simulink model "controladorpruebaio2"  (R2025a)
settings: Solver=FixedStepAuto  StartTime=0.0  StopTime=inf  FixedStep=0.015  RelTol=1e-3  EnableMultiTasking=on
libraries: px4Peripheralslib x1, px4uORBlib x1
settings Model: PacingRate=0.790000  ExtModeTrigDuration=10  Creator=The MathWorks, Inc.  LastModifiedBy=aero
settings SolverCC: AlgebraicLoopSolver=TrustRegion  PositivePriorityOrder=on  AutoInsertRateTranBlk=on  MaxZcPerStep=1.0
settings OptimizationCC: EnhancedBackFolding=on  PassReuseOutputArgsAs=Individual arguments  MaxStackSize=64  OptimizeBlockOrder=speed  DifferentSizesBufferReuse=on  OptimizationCustomize=off  EfficientTunableParamExpr=on
settings DebuggingCC: ParameterPrecisionLossMsg=none  ParameterTunabilityLossMsg=error  UnconnectedInputMsg=warning  UnconnectedOutputMsg=warning  UnconnectedLineMsg=warning  SubsystemReferenceDiagnosticForUnitTest=warning  ArithmeticOperatorsInVariantConditions=warning
settings HardwareCC: ProdBitPerPointer=32.0  ProdBitPerSizeT=32.0  ProdBitPerPtrDiffT=32.0  ProdLargestAtomicInteger=Long  ProdLargestAtomicFloat=Double  ProdWordSize=32.0  ProdLongLongMode=on  ProdHWDeviceType=ARM Compatible->ARM Cortex
settings ModelReferenceCC: EnableRefExpFcnMdlSchedulingChecks=on
settings SFSimCC: MATLABDynamicMemAlloc=off  SimTargetLang=C++  SimDLTargetLibrary=mkl-dnn
settings RTWCC: SystemTargetFile=ert.tlc  HardwareBoard=PX4 Pixhawk 6c  TLCOptions="-aInlineSetEventsForThisBaseRateFcn=TLC_FALSE -aSuppressMultiTaskScheduler=TLC_FALSE  -aRateBasedStepFcn=0"  TemplateMakefile=ert_default_tmf  GenerateReport=on  Toolchain=GNU Tools for PX4 Autopilots  IncludeHyperlinkInReport=on  LaunchReport=on  TargetLang=C++  GenerateTraceInfo=on  GenerateTraceReport=on  GenerateTraceReportSl=on  GenerateTraceReportSf=on  GenerateTraceReportEml=on  GPUComputeCapability=3.5  DLArmComputeVersion=19.05  Description=Embedded Coder
settings CodeAppCC: ForceParamTrailComments=on  IgnoreCustomStorageClasses=off  OperatorAnnotations=on  SimulinkDataObjDesc=on  SFDataObjDesc=on  InsertBlockDesc=on
settings ERTTargetCC: ExtModeTransport=3.0  ExtModeStaticAllocSize=1024.0  InlinedParameterPlacement=Hierarchical

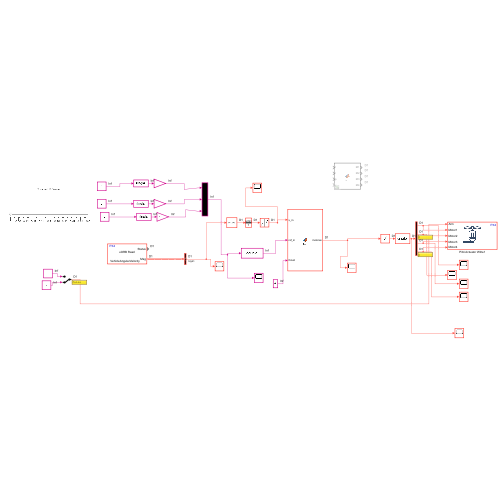
[thumbnail: Simulink's stored preview of the top-level diagram]
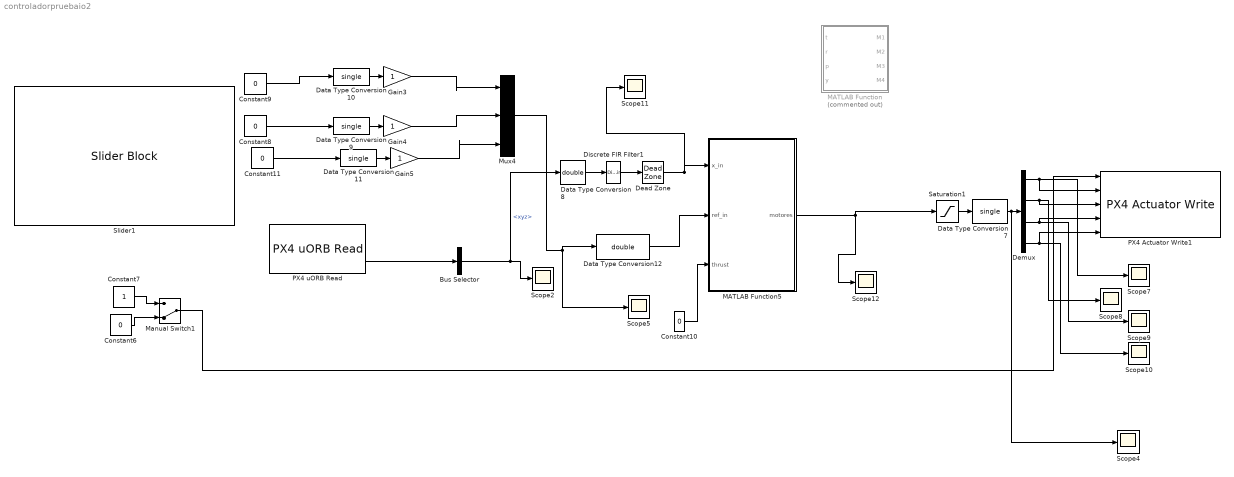
== system controladorpruebaio2 ==
  Bus Selector : BusSelector  OutputSignals=xyz
  Constant{8..11} (4 alike) : Constant  Value=0
  Constant6 : Constant  Value=0  OutDataTypeStr=boolean
  Constant7 : Constant  OutDataTypeStr=boolean
  Data Type Conversion{7,9..11} (4 alike) : DataTypeConversion  OutDataTypeStr=single  SaturateOnIntegerOverflow=off  RndMeth=Floor
  Data Type Conversion12 : DataTypeConversion  OutDataTypeStr=double  SaturateOnIntegerOverflow=off  RndMeth=Floor  LockScale=on
  Data Type Conversion8 : DataTypeConversion  OutDataTypeStr=double  SaturateOnIntegerOverflow=off  RndMeth=Floor  LockScale=on
  Dead Zone : DeadZone  LowerValue=-0.025  UpperValue=0.025
  Demux : Demux
  Discrete FIR Filter1 : DiscreteFir  Coefficients=[0.2 0.2 0.2 0.2 0.2]
  Gain3 : Gain
  Gain4 : Gain
  Gain5 : Gain
  MATLAB Function : MATLAB Function  Commented=on  TreatAsAtomicUnit=on
  MATLAB Function5 : MATLAB Function  TreatAsAtomicUnit=on
  Manual Switch1 : ManualSwitch  CurrentSetting=0
  Mux4 : Mux  Inputs=3
  PX4 Actuator Write1 : px4Peripheralslib/PX4 Actuator Write  Motor1Enable=on  Motor2Enable=on  Motor3Enable=on  Motor4Enable=on  Motor5Enable=off  Motor6Enable=off  Motor7Enable=off  Motor8Enable=off  Motor9Enable=off  Motor10Enable=off  Motor11Enable=off  Motor12Enable=off  IsMotorArray=off  Servo1Enable=off  Servo2Enable=off  Servo3Enable=off  Servo4Enable=off  Servo5Enable=off  Servo6Enable=off  Servo7Enable=off  Servo8Enable=off  IsServoArray=off
  PX4 uORB Read : px4uORBlib/PX4 uORB Read  uORBTopic=VehicleAngularVelocity  selectInstance=vehicle_angular_velocity  SampleTime=0.015  BlockingMode=off  BlockTimeout=1e-3
  Saturation1 : Saturate  UpperLimit=1  LowerLimit=0
  Scope{2,4..5,7..12} (9 alike) : Scope
      Scope10 settings: ActiveDisplayYMinimum=-0.043109886348247521  ActiveDisplayYMaximum=0.38798897713422775  DataLoggingVariableName=ScopeData10
      Scope11 settings: ActiveDisplayYMinimum=-0.15009255409240721  ActiveDisplayYMaximum=0.01667695045471191  DataLoggingVariableName=ScopeData11
      Scope12 settings: ActiveDisplayYMinimum=-1.0414258708474025  ActiveDisplayYMaximum=1.0153303161323031  DataLoggingVariableName=ScopeData12
      Scope2 settings: ActiveDisplayYMinimum=-0.33577433139146873  ActiveDisplayYMaximum=0.23733546842450437
      Scope4 settings: ActiveDisplayYMinimum=-1.5029836862276127  ActiveDisplayYMaximum=1.9132041073394161  DataLoggingVariableName=ScopeData4
      Scope5 settings: ActiveDisplayYMinimum=-1  ActiveDisplayYMaximum=1  DataLoggingVariableName=ScopeData5
      Scope7 settings: ActiveDisplayYMinimum=0.089401463046669974  ActiveDisplayYMaximum=0.69074354134500027  DataLoggingVariableName=ScopeData7
      Scope8 settings: ActiveDisplayYMinimum=-0.075780542800202952  ActiveDisplayYMaximum=0.76553872250951827  DataLoggingVariableName=ScopeData8
      Scope9 settings: ActiveDisplayYMinimum=0.00290558300912383  ActiveDisplayYMaximum=0.944020101800561  DataLoggingVariableName=ScopeData9
  Slider1 : SliderBlock  ScaleMax=0.6
  wires:
  Demux/4 -> Scope10/1, PX4 Actuator Write1/5
  Data Type Conversion8/1 -> Discrete FIR Filter1/1
  Data Type Conversion7/1 -> Scope4/1, Demux/1
  Constant6/1 -> Manual Switch1/2
  Constant9/1 -> Data Type Conversion10/1
  Gain4/1 -> Mux4/2
  Demux/3 -> Scope9/1, PX4 Actuator Write1/4
  Gain5/1 -> Mux4/3
  Mux4/1 -> Scope5/1, Data Type Conversion12/1
  PX4 uORB Read/2 -> Bus Selector/1
  Data Type Conversion12/1 -> MATLAB Function5/2(ref_in)
  Gain3/1 -> Mux4/1
  Saturation1/1 -> Data Type Conversion7/1
  Constant7/1 -> Manual Switch1/1
  Data Type Conversion9/1 -> Gain4/1
  Data Type Conversion10/1 -> Gain3/1
  Demux/1 -> Scope7/1, PX4 Actuator Write1/2
  Demux/2 -> Scope8/1, PX4 Actuator Write1/3
  MATLAB Function5/1(motores) -> Saturation1/1, Scope12/1
  Bus Selector/1 -> Scope2/1, Data Type Conversion8/1  "<xyz>"
  Data Type Conversion11/1 -> Gain5/1
  Constant8/1 -> Data Type Conversion9/1
  Constant11/1 -> Data Type Conversion11/1
  Manual Switch1/1 -> PX4 Actuator Write1/1
  Discrete FIR Filter1/1 -> Dead Zone/1
  Dead Zone/1 -> Scope11/1, MATLAB Function5/1(x_in)
  Constant10/1 -> MATLAB Function5/3(thrust)

== matlab function controladorpruebaio2/MATLAB Function ==
  data: t input; M1 output; r input; p input; y input; M2 output; M3 output; M4 output
function [M1,M2,M3,M4] = fcn(t, r, p, y)
% t: thrust
% r: roll
% p: pitch
% y: yaw

M1 = t - r - p + y;
M2 = t + r + p + y;
M3 = t + r - p - y;
M4 = t - r + p - y;

== matlab function controladorpruebaio2/MATLAB Function5 ==
  data: x_in input; motores output; ref_in input; thrust input
function motores = fcn(x_in, ref_in,thrust)
%#codegen

% --- CONFIGURACIÓN ESTÁTICA ---
persistent A B Phi F_f H  options lb ub Q_big
    
if isempty(A)
    % 1. Matrices del sistema
        A =  [   -2.0133    0.8978    6.7850;
           -0.4614    0.4367   -0.6621;
           -0.0833   -0.1459    0.3591];  
        B = [    6.0807   -2.2374   -3.6142;
            0.8163    1.1287    0.4113;
            0.1286    0.2742    0.3532];
        
    % Pre-dimensionado total (N=6, nx=3, nu=3 -> 18)
    F_mat = zeros(18, 3);
    Phi_mat = zeros(18, 18);
    Q_big_mat = zeros(18, 18);
    R_big_mat = zeros(18, 18);
    
    Q_inst = eye(3) * 1; 
    R_inst = diag([40 40 40]); 
        
    % Llenado de matrices con índices fijos para el compilador
    for i = 1:6
        row = (i-1)*3 + (1:3); % Esto es aceptado por Coder
        F_mat(row, :) = A^i;
        Q_big_mat(row, row) = Q_inst;
        R_big_mat(row, row) = R_inst;
        
        for j = 1:i
            col = (j-1)*3 + (1:3);
            Phi_mat(row, col) = A^(i-j) * B;
        end
    end
        
    H = 2 * (Phi_mat' * Q_big_mat * Phi_mat + R_big_mat);
    F_f = 2 * Phi_mat' * Q_big_mat * F_mat;
    Phi = Phi_mat; 
    Q_big = Q_big_mat;
        

           
    options = optimoptions('quadprog', 'Algorithm', 'active-set', 'Display', 'off');
    
    % Definición directa de límites
    lb = -1 * ones(18, 1); 
    ub =  1 * ones(18, 1);
end

% --- PROCESAMIENTO ---
x = double(x_in(:));
ref_vec = double(ref_in(:));


% --- LÓGICA MPC ---
U0 = zeros(18, 1); 
Ref_seq = repmat(ref_vec, 6, 1);
f = F_f * x - (2 * Phi' * Q_big * Ref_seq);
    
[U_sol, ~, exitflag] = quadprog(H, f, [], [], [], [], lb, ub, U0, options);
    
u = zeros(3,1);
if exitflag > 0
    u = U_sol(1:3);
end
    
% Mezcla final

m1= -(-u(1) + u(2) + u(3))  +thrust ;
m2= -(u(1) - u(2) + u(3))  +thrust ;
m3= -(u(1) + u(2) - u(3))  +thrust ;
m4= -(-u(1) - u(2) - u(3))  +thrust ;
motores = [m1, m2,m3,m4];
